simulink model "BehCookVat"  (R2026a)
settings: Solver=VariableStepAuto
model workspace (MAT data in the model file):
  BatchSize_bowls = 50
  CleanTime_s = 120
  DrainTime_s = 200
  FillRate_bps = 0.5
  HeaterPower_kW = 40
  HopperCap_bowls = 200
  SimmerTime_s = 1000
  VatThermalMass_JpK = 120000
undefined symbols (not defined in the file): Ambient_C, FillTemp_C, SimmerTemp_C, VAT_CLEAN, VAT_DRAIN, VAT_FILL, VAT_HEAT, VAT_IDLE, VAT_SIMMER, VatLoss_WpK
libraries: fl_lib x7, nesl_utility x5
settings Model: DataDictionary=BehParamsCommon.sldd  ParameterArgumentNames=BatchSize_bowls,HeaterPower_kW,VatThermalMass_JpK,FillRate_bps,SimmerTime_s,DrainTime_s,CleanTime_s,HopperCap_bowls  Creator=sarah  LastModifiedBy=sarah
settings SimscapeCC: SimscapeLogType=none

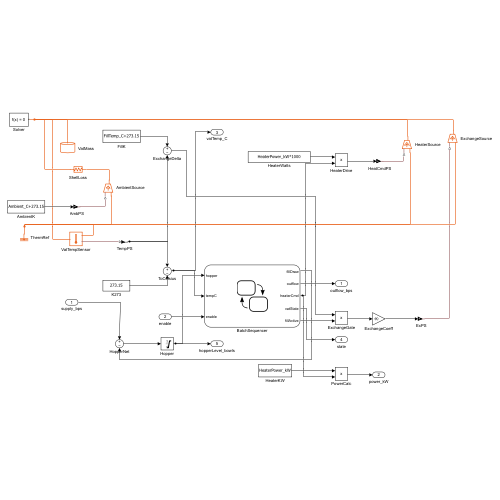
[thumbnail: Simulink's stored preview of the top-level diagram]
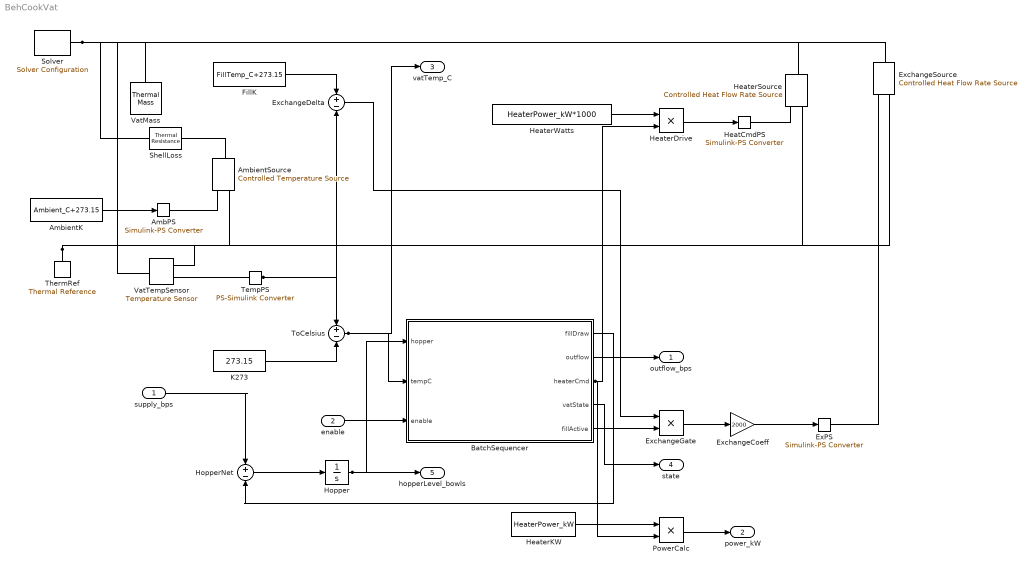
== system BehCookVat ==
  supply_bps : Inport
  enable : Inport  Port=2
  AmbPS : nesl_utility/Simulink-PS Converter  PhysicalDomain=network_engine_domain  SubClassName=ps_input  LeftPortType=input  RightPortType=output  PseudoPeriodic=off  Frequencies=[]  NoiseDistribution=none  NoiseParameters=[]  Unit=1  AffineConversion=off  FilteringAndDerivatives=provide  SimscapeFilterOrder=1  InputFilterTimeConstant=0.001  UdotUserProvided=0
  AmbientK : Constant  Value=Ambient_C+273.15
  AmbientSource : fl_lib/Thermal/Thermal Sources/Controlled Temperature Source
  BatchSequencer : Stateflow chart  TreatAsAtomicUnit=on
  ExPS : nesl_utility/Simulink-PS Converter  PhysicalDomain=network_engine_domain  SubClassName=ps_input  LeftPortType=input  RightPortType=output  PseudoPeriodic=off  Frequencies=[]  NoiseDistribution=none  NoiseParameters=[]  Unit=1  AffineConversion=off  FilteringAndDerivatives=provide  SimscapeFilterOrder=1  InputFilterTimeConstant=0.001  UdotUserProvided=0
  ExchangeCoeff : Gain  Gain=2000
  ExchangeDelta : Sum  Inputs=+-
  ExchangeGate : Product
  ExchangeSource : fl_lib/Thermal/Thermal Sources/Controlled Heat Flow Rate Source
  FillK : Constant  Value=FillTemp_C+273.15
  HeatCmdPS : nesl_utility/Simulink-PS Converter  PhysicalDomain=network_engine_domain  SubClassName=ps_input  LeftPortType=input  RightPortType=output  PseudoPeriodic=off  Frequencies=[]  NoiseDistribution=none  NoiseParameters=[]  Unit=1  AffineConversion=off  FilteringAndDerivatives=provide  SimscapeFilterOrder=1  InputFilterTimeConstant=0.001  UdotUserProvided=0
  HeaterDrive : Product
  HeaterKW : Constant  Value=HeaterPower_kW
  HeaterSource : fl_lib/Thermal/Thermal Sources/Controlled Heat Flow Rate Source
  HeaterWatts : Constant  Value=HeaterPower_kW*1000
  Hopper : Integrator  LimitOutput=on  UpperSaturationLimit=HopperCap_bowls  LowerSaturationLimit=0
  HopperNet : Sum  Inputs=+-
  K273 : Constant  Value=273.15
  PowerCalc : Product
  ShellLoss : fl_lib/Thermal/Thermal Elements/Thermal Resistance  resistance=1/VatLoss_WpK K/W  T_specify=off  T_priority=None  T=0 K  T_nominal_specify=off  T_nominal_value=1  T_nominal_unit=K  Q_specify=off  Q_priority=None  Q=0 W  Q_nominal_specify=off  Q_nominal_value=1  Q_nominal_unit=W
  Solver : nesl_utility/Solver Configuration  PhysicalDomain=network_engine_domain  SubClassName=solver  LeftPortType=input  RightPortType=generic  Tones=[]  Harmonics=[]  SimulateNoise=off  Profile=off  UseLocalSampling=off  EnableSwitchedLinearOptims=on  FrequencyDomain=off  UseCCode=off  RelTol=0.001  AbsTol=0.001  MinStep=1e-09  ToWorkspace=off  RevertToSquareIcSolve=off  NumHomotopyIterations=100  PhasorMode=off  PhasorModeNumHarmonics=1  ConsistencySolver=NEWTON_XTOL_AFTER_FTOL  CanonicalOrdering=CANONICAL  OptimizeIntermediates=OPTIMIZED  IndexReductionMethod=DerivativeReplacement  DoDC=off  ResidualTolerance=1e-09  ConsistencyTolSource=GLOBAL  ConsistencyAbsTol=0.001  ConsistencyRelTol=0.001  ConsistencyTolFactor=0.001  UseLocalSolver=off  LocalSolverChoice=NE_BACKWARD_EULER_ADVANCER  ResolveIndetEquations=on  FunctionEvalNumThread=1  LocalSolverSampleTime=0.001  DoFixedCost=off  MaxNonlinIter=3  MaxModeIter=2  ComputeImpulses=off  ImpulseIterations=2  LinearAlgebra=auto  LinearAlgebraNumThread=0  EquationFormulation=NE_TIME_EF  DelaysMemoryBudget=1024  AutomaticFiltering=on  FilteringTimeConstant=0.001  PartitionStorageMethod=AS_NEEDED  PartitionMemoryBudget=1024  PartitionMethod=ROBUST  MultibodyUseLocalSolver=off  MultibodyLocalSolverChoice=ODE1  MultibodyLocalSolverSampleTime=0.001
  TempPS : nesl_utility/PS-Simulink Converter  PhysicalDomain=network_engine_domain  SubClassName=ps_output  LeftPortType=input  RightPortType=output  PseudoPeriodic=off  Frequencies=[]  VectorFormat=inherit  Unit=inherit  AffineConversion=off
  ThermRef : fl_lib/Thermal/Thermal Elements/Thermal Reference
  ToCelsius : Sum  Inputs=+-
  VatMass : fl_lib/Thermal/Thermal Elements/Thermal Mass  mass_type=foundation.enum.constant_variable.constant  mass=VatThermalMass_JpK kg  sp_heat=1 J/(K*kg)  mass_min=1e-6 kg  num_ports=foundation.enum.numPorts2.one  m_specify=off  m_priority=High  m=1 kg  m_nominal_specify=off  m_nominal_value=1  m_nominal_unit=kg  T_specify=on  T_priority=High  T=Ambient_C+273.15 K  T_nominal_specify=off  T_nominal_value=1  T_nominal_unit=K  Q_specify=off  Q_priority=None  Q=0 W  Q_nominal_specify=off  Q_nominal_value=1  Q_nominal_unit=W
  VatTempSensor : fl_lib/Thermal/Thermal Sensors/Temperature Sensor  temperature_measure=foundation.enum.MeasurementReference.difference
  outflow_bps : Outport
  power_kW : Outport  Port=2
  vatTemp_C : Outport  Port=3
  state : Outport  Port=4
  hopperLevel_bowls : Outport  Port=5
  wires:
  BatchSequencer/1(fillDraw) -> HopperNet/2
  AmbientK/1 -> AmbPS/1
  FillK/1 -> ExchangeDelta/1
  supply_bps/1 -> HopperNet/1
  TempPS/1 -> ExchangeDelta/2, ToCelsius/1
  K273/1 -> ToCelsius/2
  HopperNet/1 -> Hopper/1
  ExchangeCoeff/1 -> ExPS/1
  ExchangeDelta/1 -> ExchangeGate/1
  ToCelsius/1 -> BatchSequencer/2(tempC), vatTemp_C/1
  enable/1 -> BatchSequencer/3(enable)
  BatchSequencer/3(heaterCmd) -> PowerCalc/2, HeaterDrive/2
  Hopper/1 -> BatchSequencer/1(hopper), hopperLevel_bowls/1
  HeaterWatts/1 -> HeaterDrive/1
  PowerCalc/1 -> power_kW/1
  BatchSequencer/2(outflow) -> outflow_bps/1
  BatchSequencer/4(vatState) -> state/1
  BatchSequencer/5(fillActive) -> ExchangeGate/2
  HeaterKW/1 -> PowerCalc/1
  HeaterDrive/1 -> HeatCmdPS/1
  ExchangeGate/1 -> ExchangeCoeff/1
  connections:
  Solver/RConn1 -- VatMass/LConn1 -- ExchangeSource/LConn1 -- HeaterSource/LConn1 -- ShellLoss/LConn1 -- VatTempSensor/LConn1
  ExPS/RConn1 -- ExchangeSource/RConn1
  AmbPS/RConn1 -- AmbientSource/RConn1
  ThermRef/LConn1 -- VatTempSensor/RConn1 -- HeaterSource/RConn2 -- ExchangeSource/RConn2 -- AmbientSource/RConn2
  ShellLoss/RConn1 -- AmbientSource/LConn1
  VatTempSensor/RConn2 -- TempPS/LConn1
  HeatCmdPS/RConn1 -- HeaterSource/RConn1

== stateflow chart BehCookVat/BatchSequencer ==
  settings: updateMethod=DISCRETE  sampleTime=1
  state Idle
    du: fillDraw = 0; outflow = 0; heaterCmd = 0; fillActive = 0; vatState = VAT_IDLE;
  state Fill
    du: fillDraw = FillRate_bps; outflow = 0; heaterCmd = 0; fillActive = 1; vatState = VAT_FILL;
  state Heat
    du: fillDraw = 0; outflow = 0; heaterCmd = 1; fillActive = 0; vatState = VAT_HEAT;
  state Simmer
    du: fillDraw = 0; outflow = 0; heaterCmd = double(tempC < SimmerTemp_C); fillActive = 0; vatState = VAT_SIMMER;
  state Drain
    du: fillDraw = 0; outflow = BatchSize_bowls/DrainTime_s; heaterCmd = 0; fillActive = 0; vatState = VAT_DRAIN;
  state Clean
    du: fillDraw = 0; outflow = 0; heaterCmd = 0; fillActive = 0; vatState = VAT_CLEAN;
  (default) -> Idle
  Clean -> Idle : [after(CleanTime_s, sec)]
  Simmer -> Idle [order 1] : [enable < 0.5]
  Heat -> Idle [order 1] : [enable < 0.5]
  Idle -> Fill : [enable > 0.5 && hopper >= BatchSize_bowls]
  Fill -> Idle [order 1] : [enable < 0.5]
  Fill -> Heat [order 2] : [after(BatchSize_bowls/FillRate_bps, sec)]
  Heat -> Simmer [order 2] : [tempC >= SimmerTemp_C]
  Simmer -> Drain [order 2] : [after(SimmerTime_s, sec)]
  Drain -> Clean : [after(DrainTime_s, sec)]
  data: hopper input double; tempC input double; enable input double; fillDraw output double; outflow output double; heaterCmd output double; vatState output uint8; fillActive output double; BatchSize_bowls parameter double; FillRate_bps parameter double; SimmerTime_s parameter double; DrainTime_s parameter double; CleanTime_s parameter double; SimmerTemp_C parameter double; VAT_IDLE parameter uint8; VAT_FILL parameter uint8; VAT_HEAT parameter uint8; VAT_SIMMER parameter uint8; VAT_DRAIN parameter uint8; VAT_CLEAN parameter uint8
